simulink model "simlinkdatei"  (Simulink 7.9)
settings: Solver=ode45  StartTime=0.0  StopTime=10.0  RelTol=1e-3
settings Model: Creator=s67750  LastModifiedBy=s67750

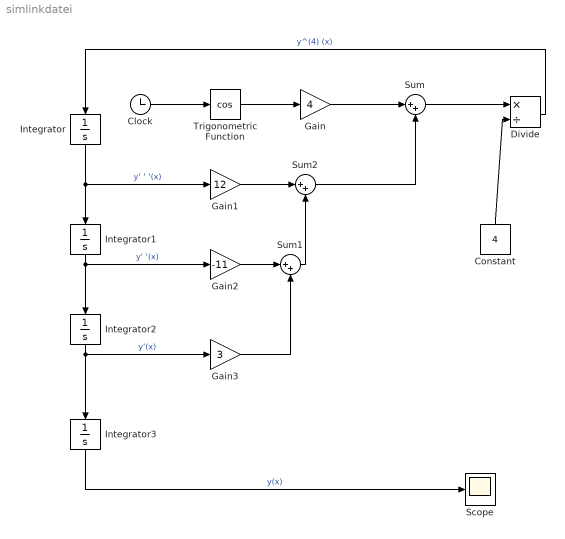
== system simlinkdatei ==
  Clock : Clock
  Constant : Constant  Value=4
  Divide : Product  Inputs=*/
  Gain : Gain  Gain=4
  Gain1 : Gain  Gain=12
  Gain2 : Gain  Gain=-11
  Gain3 : Gain  Gain=3
  Integrator : Integrator  InitialCondition=2
  Integrator1 : Integrator  InitialCondition=3
  Integrator2 : Integrator  InitialCondition=4
  Integrator3 : Integrator  InitialCondition=5
  Scope : Scope
  Sum : Sum  Inputs=|++
  Sum1 : Sum  Inputs=|++
  Sum2 : Sum  Inputs=|++
  Trigonometric Function : Trigonometry  Operator=cos
  wires:
  Integrator/1 -> Integrator1/1, Gain1/1  "y' ' '(x)"
  Integrator1/1 -> Integrator2/1, Gain2/1  "y' '(x)"
  Integrator2/1 -> Integrator3/1, Gain3/1  "y'(x)"
  Integrator3/1 -> Scope/1  "y(x)"
  Gain3/1 -> Sum1/2
  Gain2/1 -> Sum1/1
  Sum1/1 -> Sum2/2
  Gain1/1 -> Sum2/1
  Divide/1 -> Integrator/1  "y^(4) (x)"
  Clock/1 -> Trigonometric Function/1
  Trigonometric Function/1 -> Gain/1
  Sum2/1 -> Sum/2
  Gain/1 -> Sum/1
  Constant/1 -> Divide/2
  Sum/1 -> Divide/1
